simulink model "s_track_model"  (R2021b)
settings: Solver=VariableStepAuto  StartTime=0.0  StopTime=10  FixedStep=dt_sim  RelTol=1e-3  EnableMultiTasking=on
values from neighbouring files (symbols this model uses):
  A_sim = [(-CF-CR)/(m*Vv),(-CF*a+CR*b-m*Vv^2)/(m*Vv^2) ... (first row only)    [s_track_ini.m]
  ay_max = 10    [s_track_ini.m]
  B_sim = [CF/(m*Vv) CR/(m*Vv) ... (first row only)    [s_track_ini.m]
  beta_max = 80    [s_track_ini.m]
  C_sim = [1,0 ... (first row only)    [s_track_ini.m]
  D_sim = [0 0 ... (first row only)    [s_track_ini.m]
  dvol_max = 5    [s_track_ini.m]
  sel_man = 1    [s_track_ini.m]
  tau_s = 15    [s_track_ini.m]
  V = V/3.6    (= 27.7777777778)    [s_track_ini.m]
  x_0 = -62.1916    [s_track_ini.m]
  y_0 = -134.804    [s_track_ini.m]
libraries: simulink x15, simulink_extras x8, sim3dcameralib x1, sim3dlib x1, sim3dautolib x1, dspvision x1
settings Model: Creator=gianl  LastModifiedBy=asdas
settings SolverCC: AlgebraicLoopSolver=TrustRegion
settings DataIOCC: ReturnWorkspaceOutputsName=out_SLX
settings OptimizationCC: LifeSpan=1
settings DebuggingCC: SFExecutionAtInitializationDiag=none  SFMachineParentedDataDiag=warning  ArithmeticOperatorsInVariantConditions=warning
settings SFSimCC: SimUseLocalCustomCode=off  CustomCodeUndefinedFunction=UseInterfaceOnly
settings RTWCC: RTWUseLocalCustomCode=off
settings CodeAppCC: StateflowObjectComments=on

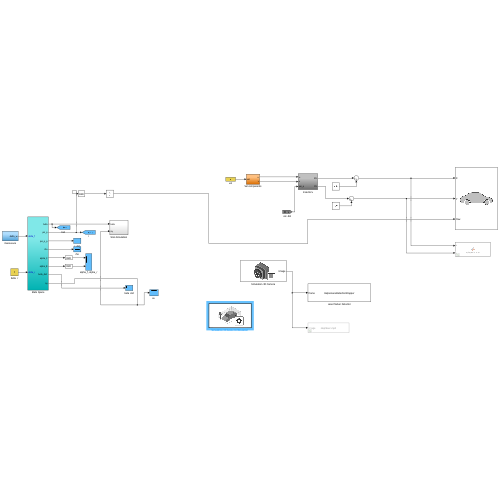
[thumbnail: Simulink's stored preview of the top-level diagram]
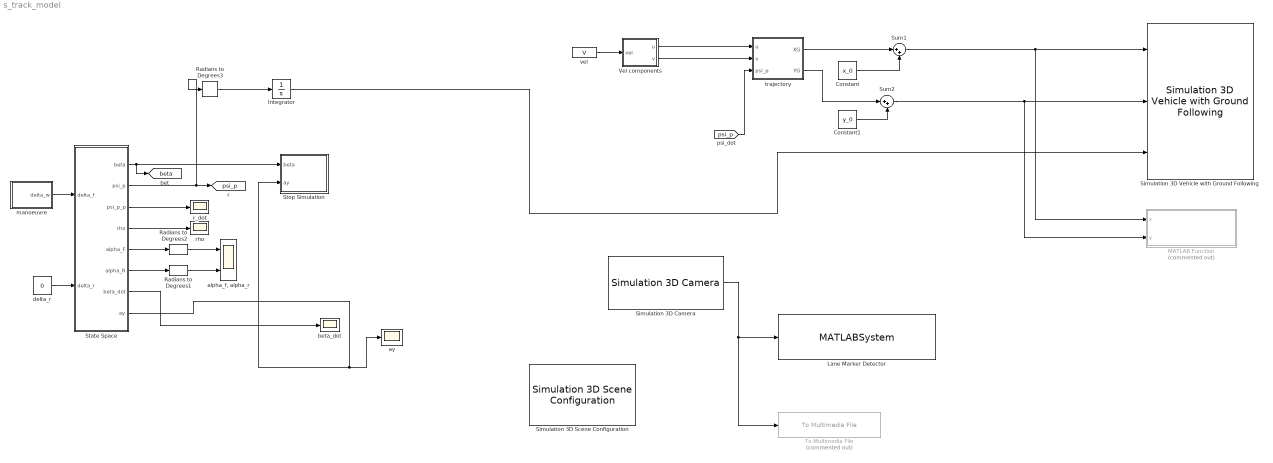
== system s_track_model ==
  Constant : Constant  Value=x_0
  Constant1 : Constant  Value=y_0
  Integrator : Integrator
  Lane Marker Detector : MATLABSystem  System=HelperLaneDetectorWrapper  EnableLaneTracker=on  EnableDisplays=on  Camera=Camera  SimulateUsing=Interpreted execution
      mask Type: HelperLaneDetectorWrapper
      mask Display:
      | disp('HelperLaneDetectorWrapper');
      | port_label('input',1,'frame');
  MATLAB Function : MATLAB Function  Commented=on  TreatAsAtomicUnit=on
      settings: ModelCloseFcn=|
      | % Find figure with name "Scene Display"
      | hFig = findobj('Type', 'figure', 'Name', 'Scene Display');
      | 
      | if ~isempty(hFig) && isvalid(hFig)
      |     close(hFig);
      | end
      | clear hFig;
  Radians to Degrees1 : simulink_extras/Transformations/Radians to Degrees
  Radians to Degrees2 : simulink_extras/Transformations/Radians to Degrees
  Radians to Degrees3 : simulink_extras/Transformations/Radians to Degrees
  Simulation 3D Camera : sim3dcameralib/Simulation 3D Camera  sensorTag=Sim3dSensor1  sensorId=1  sensorName=Sim3dSensor1  vehTagList={'Scene Origin';'SimulinkVehicle1'}  vehTag=SimulinkVehicle1  mountLoc=Rearview mirror  offsetFlag=off  tmountOffset=[0, 0, 0]  extTmount=off  rmountOffset=[0, 0, 0]  extRmount=off  FocalLength=[320, 320]  OpticalCenter=[640, 480]/2  ImageSize=[480, 640]  RadialDistortion=[0, 0]  TangentialDistortion=[0, 0]  SensorSkew=0  DepthOutportEnabled=off  SemanticOutportEnabled=off  TransformOutportEnabled=off  SampleTime=-1  mountPoint=[0.319999992847443 0 1.19000005722046]  mountOrientation=[0 0 0]  aMode=3  ID=1
      settings: SourceProductBaseCode=AE,DR,UV,VE
  Simulation 3D Scene Configuration : sim3dlib/Simulation 3D Scene Configuration  Priority=0  ProjectFormat_internal=Default Scenes  ProjectFormat=Default Scenes  SceneDesc=Straight road  ProjectName=C:\Program Files\MATLAB\R2021b\toolbox\shared\sim3d_projects\automotive_project\UE4\WindowsNoEditor\VehicleSimulation.exe  ScenePath=/Game/Maps/HwStrght  vehTagList={'Scene Origin';'SimulinkVehicle1'}  vehTag=SimulinkVehicle1  OpVisEn=off  Ts=1/60  EnableWindow=off  EnableWeather=off  SunAltitude=40.0  SunAzimuth=90  clouds=10  wind=1  fog=0  rain=0  sensorTag=MainCamera1  sensorId=1  sensorName=MainCamera1  mountLoc=Origin  offsetFlag=off  tmountOffset=[0, 0, 0]  rmountOffset=[0, 0, 0]  HorizontalResolution=1280  VerticalResolution=720  HorizontalFOV=60  mountPoint=[0 0 0]  mountOrientation=[0 0 0]  aMode=3  ID=1
      settings: SourceProductBaseCode=AE,DR,UV,VE
  Simulation 3D Vehicle with Ground Following : sim3dautolib/Simulation 3D Vehicle with Ground Following  Priority=-1  PassVehMesh=Muscle car  PassVehMesh_Internal=Muscle car  MeshPath=/MathWorksSimulation/Vehicles/Muscle/Meshes/SK_MuscleCar.SK_MuscleCar  TrackWidth=1.9  WheelBase=3  WheelRadius=0.35  VehColor=Red  VehColor_Internal=Red  InitialPos=[0,0,0]  InitialRot=[0, 0, 0]  ActorName=SimulinkVehicle1  SampleTime=-1  ActorType=SimulinkVehicle  ID=1  aMode=3  ActorTag=SimulinkVehicle1  CoordinateScheme=ISO  VehLightsControl=off  HeadlightColor=[ 1, 1, 1 ]  HighBeamIntensity=100000  LowBeamIntensity=60000  HighBeamConeAngle=70  LowBeamConeAngle=70  LeftHeadlightOrientation=[ 0, 0 ]  RightHeadlightOrientation=[ 0, 0 ]  BrakelightIntensity=500  ReverselightIntensity=500  SignallightIntensity=500  SignallightPeriod=1  SignalPulseWidth=50  TransformOutportEnabled=off
      settings: SourceProductBaseCode=AE,DR,UV,VE
  State Space : Subsystem
  Stop Simulation : Subsystem
  Sum1 : Sum  Inputs=|++
  Sum2 : Sum  Inputs=|++
  To Multimedia File : dspvision/To Multimedia File  Commented=on  outputFilename=stepSteer.mp4  streamSelection=Video only  videoCompressor=None (uncompressed)  audioCompressor=None (uncompressed)  imagePorts=One multidimensional signal  fileType=MPEG4  audioDatatype=Determine from input data type  fourcc=RGB  videoQuality=75  mj2000CompFactor=10
  Vel components : Subsystem
  "alpha_f, alpha_r" : Scope  NumInputPorts=2
  "ay " : Scope
  beta_dot : Scope
  delta_r : Constant  Value=0
  manoeuvre : Subsystem
  r_dot : Scope
  rho : Scope
  trajectory : Subsystem
  vel : Constant  Value=V
  tag scope: beta=global, psi_p=global
  wires:
  manoeuvre/1(delta_w) -> State Space/1(delta_f)
  State Space/1(beta) -> [beta], Stop Simulation/1(beta)
  State Space/2(psi_p) -> Radians to Degrees3/1, [psi_p]
  State Space/3(psi_p_p) -> r_dot/1
  vel/1 -> Vel components/1(vel)
  Vel components/1(u) -> trajectory/1(u)
  Vel components/2(v) -> trajectory/2(v)
  [psi_p] -> trajectory/3(psi_p)
  State Space/4(rho) -> rho/1
  State Space/5(alpha_F) -> Radians to Degrees2/1
  State Space/6(alpha_R) -> Radians to Degrees1/1
  Sum1/1 -> MATLAB Function/1(x), Simulation 3D Vehicle with Ground Following/1
  Sum2/1 -> MATLAB Function/2(y), Simulation 3D Vehicle with Ground Following/2
  delta_r/1 -> State Space/2(delta_r)
  State Space/7("beta_dot ") -> beta_dot/1
  State Space/8(ay) -> "ay "/1, Stop Simulation/2(ay)
  Radians to Degrees2/1 -> "alpha_f, alpha_r"/1
  Radians to Degrees1/1 -> "alpha_f, alpha_r"/2
  Simulation 3D Camera/1 -> To Multimedia File/1, Lane Marker Detector/1
  Integrator/1 -> Simulation 3D Vehicle with Ground Following/3
  Radians to Degrees3/1 -> Integrator/1
  trajectory/1(XG) -> Sum1/1
  Constant/1 -> Sum1/2
  trajectory/2(YG) -> Sum2/1
  Constant1/1 -> Sum2/2

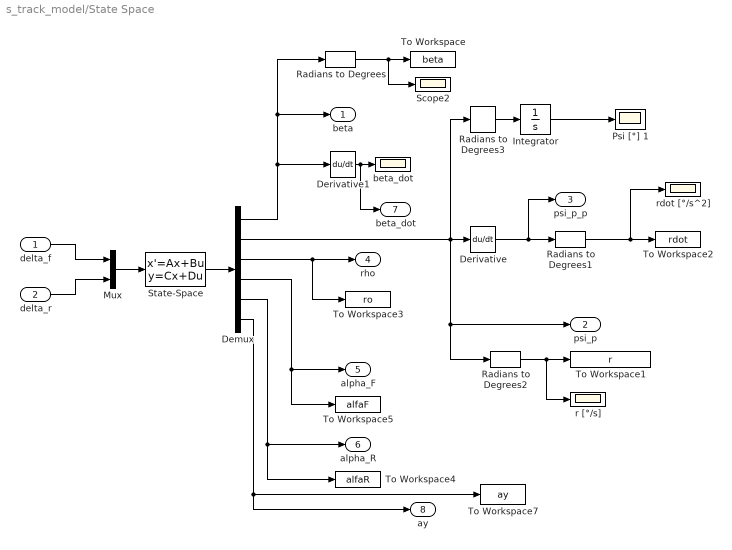
== system s_track_model/State Space ==
  delta_f : Inport
  delta_r : Inport  Port=2
  Demux : Demux  Outputs=6
  Derivative : Derivative
  Derivative1 : Derivative
  Integrator : Integrator
  Mux : Mux  Inputs=2
  Psi [°] 1 : Scope
  Radians to Degrees{,1..3} (4 alike) : simulink_extras/Transformations/Radians to Degrees
  Scope2 : Scope
  State-Space : StateSpace  A=A_sim  B=B_sim  C=C_sim  D=D_sim  InitialCondition=[0 0]  ContinuousStateAttributes={'sideslip_angle','yaw_rate'}
  To Workspace : ToWorkspace  VariableName=beta  SaveFormat=Timeseries  SampleTime=-1
  To Workspace1 : ToWorkspace  VariableName=r  SaveFormat=Timeseries  SampleTime=-1
  To Workspace2 : ToWorkspace  VariableName=rdot  SaveFormat=Timeseries  SampleTime=-1
  To Workspace3 : ToWorkspace  VariableName=ro  SaveFormat=Timeseries  SampleTime=-1
  To Workspace4 : ToWorkspace  VariableName=alfaR  SaveFormat=Timeseries  SampleTime=-1
  To Workspace5 : ToWorkspace  VariableName=alfaF  SaveFormat=Timeseries  SampleTime=-1
  To Workspace7 : ToWorkspace  VariableName=ay  SaveFormat=Timeseries  SampleTime=-1
      settings: Save2DSignal=2-D array (concatenate along first dimension)
  beta_dot : Scope
  r [°/s] : Scope
  rdot [°/s^2] : Scope
  beta : Outport  VectorParamsAs1DForOutWhenUnconnected=off
  psi_p : Outport  Port=2  VectorParamsAs1DForOutWhenUnconnected=off
  psi_p_p : Outport  Port=3  VectorParamsAs1DForOutWhenUnconnected=off
  rho : Outport  Port=4  VectorParamsAs1DForOutWhenUnconnected=off
  alpha_F : Outport  Port=5  VectorParamsAs1DForOutWhenUnconnected=off
  alpha_R : Outport  Port=6  VectorParamsAs1DForOutWhenUnconnected=off
  "beta_dot " : Outport  Port=7  VectorParamsAs1DForOutWhenUnconnected=off
  ay : Outport  Port=8  VectorParamsAs1DForOutWhenUnconnected=off
  wires:
  Demux/2 -> psi_p/1, Radians to Degrees2/1, Radians to Degrees3/1, Derivative/1
  Demux/1 -> Derivative1/1, beta/1, Radians to Degrees/1
  State-Space/1 -> Demux/1
  Derivative/1 -> Radians to Degrees1/1, psi_p_p/1
  Radians to Degrees/1 -> Scope2/1, To Workspace/1
  Radians to Degrees1/1 -> rdot [°/s^2]/1, To Workspace2/1
  Radians to Degrees2/1 -> r [°/s]/1, To Workspace1/1
  Demux/3 -> To Workspace3/1, rho/1
  Demux/4 -> alpha_F/1, To Workspace5/1
  Demux/5 -> To Workspace4/1, alpha_R/1
  Radians to Degrees3/1 -> Integrator/1
  Integrator/1 -> Psi [°] 1/1
  Derivative1/1 -> "beta_dot "/1, beta_dot/1
  delta_f/1 -> Mux/1
  Mux/1 -> State-Space/1
  delta_r/1 -> Mux/2
  Demux/6 -> ay/1, To Workspace7/1

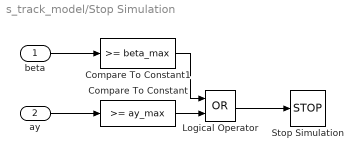
== system s_track_model/Stop Simulation ==
  beta : Inport
  ay : Inport  Port=2
  Compare To Constant : simulink/Logic and Bit Operations/Compare To Constant  relop=>=  const=ay_max  OutDataTypeStr=boolean
  Compare To Constant1 : simulink/Logic and Bit Operations/Compare To Constant  relop=>=  const=beta_max  OutDataTypeStr=boolean
  Logical Operator : Logic  Operator=OR  AllPortsSameDT=off  OutDataTypeStr=boolean
  Stop Simulation : Stop
  wires:
  Logical Operator/1 -> Stop Simulation/1
  ay/1 -> Compare To Constant/1
  beta/1 -> Compare To Constant1/1
  Compare To Constant/1 -> Logical Operator/2
  Compare To Constant1/1 -> Logical Operator/1

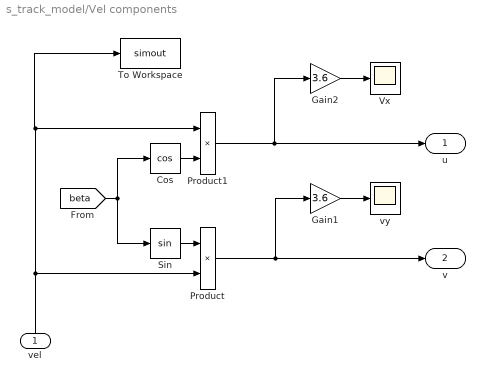
== system s_track_model/Vel components ==
  vel : Inport
  Cos : Trigonometry  Operator=cos
  Gain1 : Gain  Gain=3.6
  Gain2 : Gain  Gain=3.6
  Product : Product
  Product1 : Product
  Sin : Trigonometry
  To Workspace : ToWorkspace  VariableName=simout  SaveFormat=Timeseries  SampleTime=-1
  Vx : Scope
  vy : Scope
  u : Outport  VectorParamsAs1DForOutWhenUnconnected=off
  v : Outport  Port=2  VectorParamsAs1DForOutWhenUnconnected=off
  wires:
  Product/1 -> Gain1/1, v/1
  vel/1 -> Product/2, Product1/1, To Workspace/1
  Gain1/1 -> vy/1
  Gain2/1 -> Vx/1
  Cos/1 -> Product1/2
  Product1/1 -> Gain2/1, u/1
  [beta] -> Sin/1, Cos/1
  Sin/1 -> Product/1

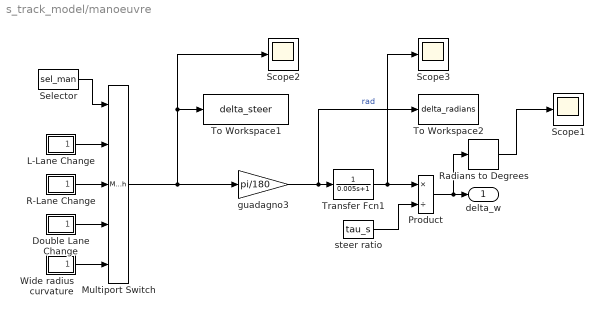
== system s_track_model/manoeuvre ==
  Double Lane Change : Subsystem
  L-Lane Change : Subsystem
  Multiport Switch : MultiPortSwitch  Inputs=4
  Product : Product  Inputs=*/  RndMeth=Zero
  R-Lane Change : Subsystem
  Radians to Degrees : simulink_extras/Transformations/Radians to Degrees
  Scope1 : Scope
  Scope2 : Scope
  Scope3 : Scope
  Selector : Constant  Value=sel_man
  To Workspace1 : ToWorkspace  VariableName=delta_steer  SaveFormat=Timeseries  SampleTime=-1
  To Workspace2 : ToWorkspace  VariableName=delta_radians  SaveFormat=Timeseries  SampleTime=-1
  Transfer Fcn1 : TransferFcn  Denominator=[0.005 1]
  Wide radius curvature : Subsystem
  guadagno3 : Gain  Gain=pi/180  SaturateOnIntegerOverflow=on  OutDataTypeStr=Inherit: Same as input  ParamDataTypeStr=Inherit: Same as input
  "steer ratio " : Constant  Value=tau_s
  delta_w : Outport  VectorParamsAs1DForOutWhenUnconnected=off
  wires:
  Selector/1 -> Multiport Switch/1
  L-Lane Change/1(delta) -> Multiport Switch/2
  Multiport Switch/1 -> guadagno3/1, To Workspace1/1, Scope2/1
  guadagno3/1 -> To Workspace2/1, Transfer Fcn1/1  "rad"
  "steer ratio "/1 -> Product/2
  Product/1 -> Radians to Degrees/1, delta_w/1
  Transfer Fcn1/1 -> Scope3/1, Product/1
  Double Lane Change/1(delta) -> Multiport Switch/4
  Wide radius curvature/1(delta) -> Multiport Switch/5
  Radians to Degrees/1 -> Scope1/1
  R-Lane Change/1(delta) -> Multiport Switch/3

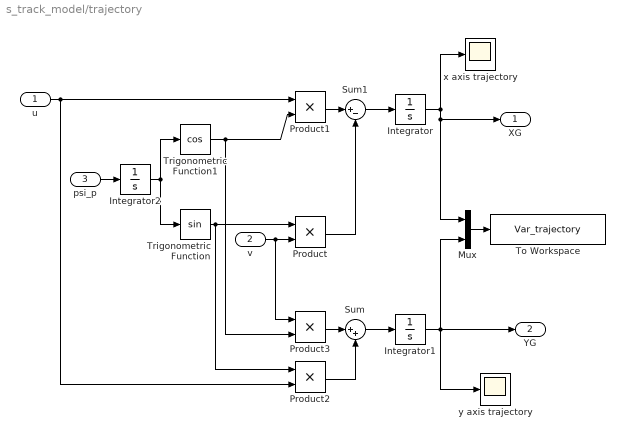
== system s_track_model/trajectory ==
  u : Inport
  v : Inport  Port=2
  psi_p : Inport  Port=3
  Integrator : Integrator
  Integrator1 : Integrator
  Integrator2 : Integrator
  Mux : Mux  Inputs=2
  Product{,1..3} (4 alike) : Product  InputSameDT=on  SaturateOnIntegerOverflow=on  OutDataTypeStr=Inherit: Same as first input
  Sum : Sum  Inputs=|++  InputSameDT=on  SaturateOnIntegerOverflow=on  OutDataTypeStr=Inherit: Same as first input
  Sum1 : Sum  Inputs=|+-  InputSameDT=on  SaturateOnIntegerOverflow=on  OutDataTypeStr=Inherit: Same as first input
  To Workspace : ToWorkspace  VariableName=Var_trajectory  SampleTime=-1
      settings: Save2DSignal=2-D array (concatenate along first dimension)
      settings: InitFcn=|
      | ParentName = get_param(gcb,'Parent');
      | cont = max(find(ParentName=='/'));
      | set_param(gcb,'VariableName',strcat('Var_',ParentName(cont+1:length(ParentName))));
      | clear ParentName cont
  Trigonometric Function : Trigonometry
  Trigonometric Function1 : Trigonometry  Operator=cos
  x axis trajectory : Scope
  y axis trajectory : Scope
  XG : Outport  VectorParamsAs1DForOutWhenUnconnected=off
  YG : Outport  Port=2  VectorParamsAs1DForOutWhenUnconnected=off
  wires:
  psi_p/1 -> Integrator2/1
  Product1/1 -> Sum1/1
  Product/1 -> Sum1/2
  Sum1/1 -> Integrator/1
  Trigonometric Function/1 -> Product/1, Product2/1
  u/1 -> Product2/2, Product1/1
  v/1 -> Product/2, Product3/1
  Trigonometric Function1/1 -> Product1/2, Product3/2
  Product3/1 -> Sum/1
  Product2/1 -> Sum/2
  Sum/1 -> Integrator1/1
  Integrator/1 -> XG/1, Mux/1, x axis trajectory/1
  Integrator1/1 -> YG/1, y axis trajectory/1, Mux/2
  Mux/1 -> To Workspace/1
  Integrator2/1 -> Trigonometric Function/1, Trigonometric Function1/1

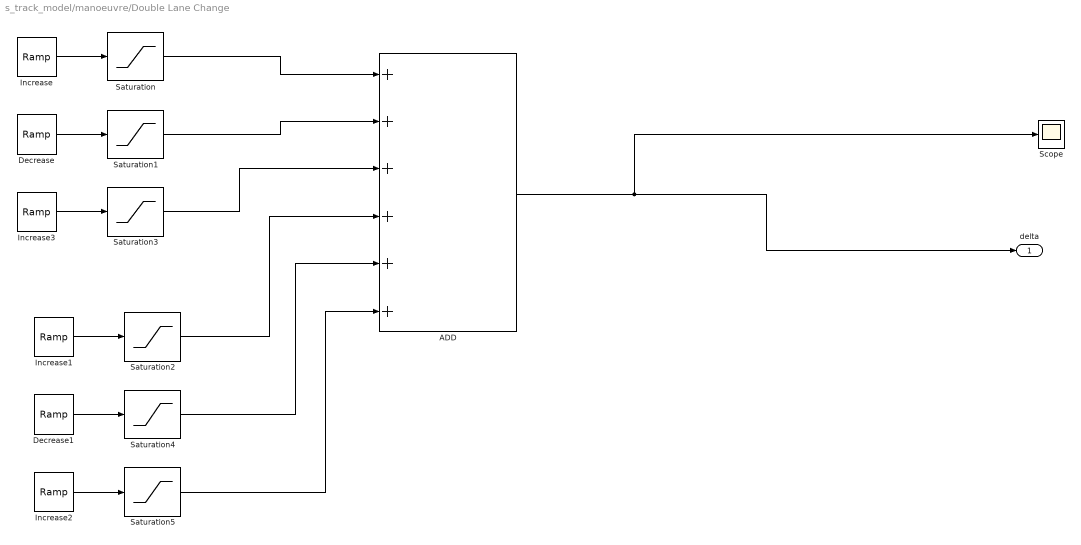
== system s_track_model/manoeuvre/Double Lane Change ==
  ADD : Sum  Inputs=++++++
  Decrease : simulink/Sources/Ramp  slope=-400  start=2.2  InitialOutput=0
  Decrease1 : simulink/Sources/Ramp  slope=400  start=6.7  InitialOutput=0
  Increase : simulink/Sources/Ramp  slope=400  start=0.5  InitialOutput=0
  Increase1 : simulink/Sources/Ramp  slope=-400  start=5  InitialOutput=0
  Increase2 : simulink/Sources/Ramp  slope=-400  start=8.4  InitialOutput=0
  Increase3 : simulink/Sources/Ramp  slope=400  start=3.9  InitialOutput=0
  Saturation : Saturate  UpperLimit=dvol_max  LowerLimit=0
  Saturation1 : Saturate  UpperLimit=0  LowerLimit=-2*dvol_max
  Saturation2 : Saturate  UpperLimit=0  LowerLimit=-dvol_max
  Saturation3 : Saturate  UpperLimit=dvol_max  LowerLimit=0
  Saturation4 : Saturate  UpperLimit=2*dvol_max  LowerLimit=0
  Saturation5 : Saturate  UpperLimit=0  LowerLimit=-dvol_max
  Scope : Scope
  delta : Outport  InitialOutput=0  VectorParamsAs1DForOutWhenUnconnected=off
  wires:
  Increase/1 -> Saturation/1
  Decrease/1 -> Saturation1/1
  Increase3/1 -> Saturation3/1
  Saturation/1 -> ADD/1
  Saturation1/1 -> ADD/2
  Saturation3/1 -> ADD/3
  Saturation4/1 -> ADD/5
  Increase2/1 -> Saturation5/1
  Saturation5/1 -> ADD/6
  Increase1/1 -> Saturation2/1
  Saturation2/1 -> ADD/4
  Decrease1/1 -> Saturation4/1
  ADD/1 -> Scope/1, delta/1

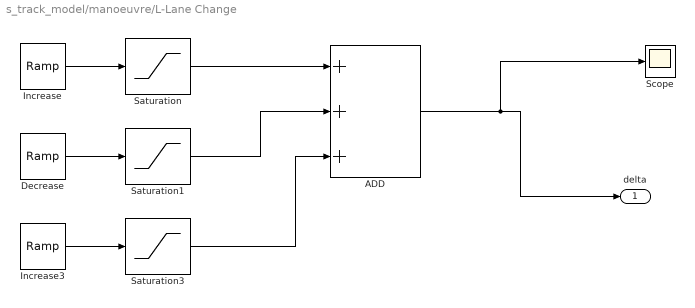
== system s_track_model/manoeuvre/L-Lane Change ==
  ADD : Sum  Inputs=+++
  Decrease : simulink/Sources/Ramp  slope=-400  start=2.2  InitialOutput=0
  Increase : simulink/Sources/Ramp  slope=400  start=0.5  InitialOutput=0
  Increase3 : simulink/Sources/Ramp  slope=400  start=3.9  InitialOutput=0
  Saturation : Saturate  UpperLimit=dvol_max  LowerLimit=0
  Saturation1 : Saturate  UpperLimit=0  LowerLimit=-2*dvol_max
  Saturation3 : Saturate  UpperLimit=dvol_max  LowerLimit=0
  Scope : Scope
  delta : Outport  InitialOutput=0  VectorParamsAs1DForOutWhenUnconnected=off
  wires:
  Increase/1 -> Saturation/1
  Saturation/1 -> ADD/1
  Saturation3/1 -> ADD/3
  ADD/1 -> Scope/1, delta/1
  Saturation1/1 -> ADD/2
  Decrease/1 -> Saturation1/1
  Increase3/1 -> Saturation3/1

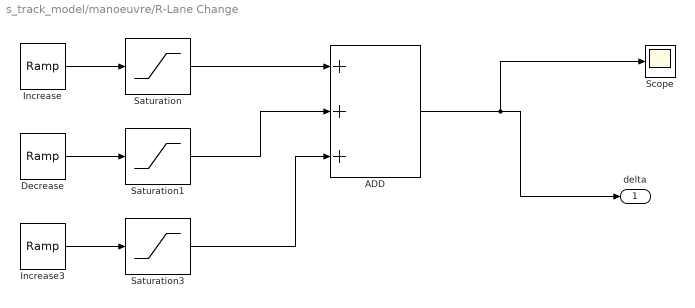
== system s_track_model/manoeuvre/R-Lane Change ==
  ADD : Sum  Inputs=+++
  Decrease : simulink/Sources/Ramp  slope=400  start=2  InitialOutput=0
  Increase : simulink/Sources/Ramp  slope=-400  start=0.5  InitialOutput=0
  Increase3 : simulink/Sources/Ramp  slope=-400  start=3.5  InitialOutput=0
  Saturation : Saturate  UpperLimit=0  LowerLimit=-dvol_max
  Saturation1 : Saturate  UpperLimit=2*dvol_max  LowerLimit=0
  Saturation3 : Saturate  UpperLimit=0  LowerLimit=-dvol_max
  Scope : Scope
  delta : Outport  InitialOutput=0  VectorParamsAs1DForOutWhenUnconnected=off
  wires:
  Saturation1/1 -> ADD/2
  Increase3/1 -> Saturation3/1
  Saturation/1 -> ADD/1
  ADD/1 -> Scope/1, delta/1
  Saturation3/1 -> ADD/3
  Decrease/1 -> Saturation1/1
  Increase/1 -> Saturation/1

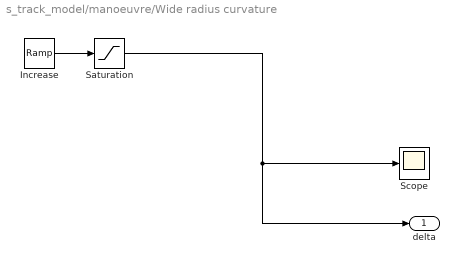
== system s_track_model/manoeuvre/Wide radius curvature ==
  Increase : simulink/Sources/Ramp  slope=400  start=1  InitialOutput=0
  Saturation : Saturate  UpperLimit=dvol_max  LowerLimit=0
  Scope : Scope
  delta : Outport  VectorParamsAs1DForOutWhenUnconnected=off
  wires:
  Increase/1 -> Saturation/1
  Saturation/1 -> delta/1, Scope/1

== matlab function s_track_model/MATLAB Function ==
  settings: updateMethod=DISCRETE  sampleTime=.02
  data: x input; y input
function helperPlotPath(x, y)
%helperPlotPath Plot path on scene image
%   helperPlotPath plots the path specified by x,y waypoint on the current
%   scene.

% Copyright 2019 The MathWorks, Inc.

coder.extrinsic('helperGetCurrentScene', 'helperShowSceneImage', ...
    'figure','movegui','isvalid','images.roi.Polyline',...
    'helperUpdatePolyline');

persistent hFig hPoly;

if isempty(hFig)
    % Query the model to find the scene selection
    sceneName = helperGetCurrentScene();
    
    % Create a figure and display the scene on it
    hFig = figure('Name', 'Scene Display');
    helperShowSceneImage(sceneName);
    
    % Move figure to right of screen
    movegui(hFig, 'east')
    
    % Display the path
    hold on
    hPoly = images.roi.Polyline('Parent', gca, 'Position', [x y], 'InteractionsAllowed', 'none');
end

if isvalid(hFig)
    % Update the path with the new point
    helperUpdatePolyline(hPoly, x, y);
end
end
